simulink model "LQR"  (R2024a)
settings: Solver=ode4  StartTime=0.0  StopTime=simtime  FixedStep=0.1  RelTol=1e-3
values from neighbouring files (symbols this model uses):
  C = [1 0 0 0 0 0 -1 0 0 0 0 0 ... (45 elements, 5x9)]    [C.mat]
undefined symbols (not defined in the file or in its folder): Ki, Kp, syys
settings Model: Creator=soeta  LastModifiedBy=soeta
settings DataIOCC: ReturnWorkspaceOutputs=off

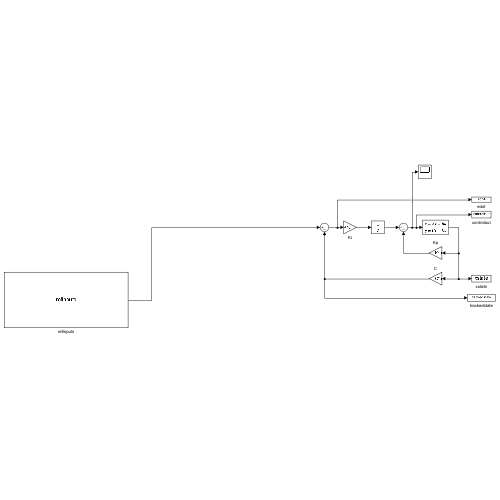
[thumbnail: Simulink's stored preview of the top-level diagram]
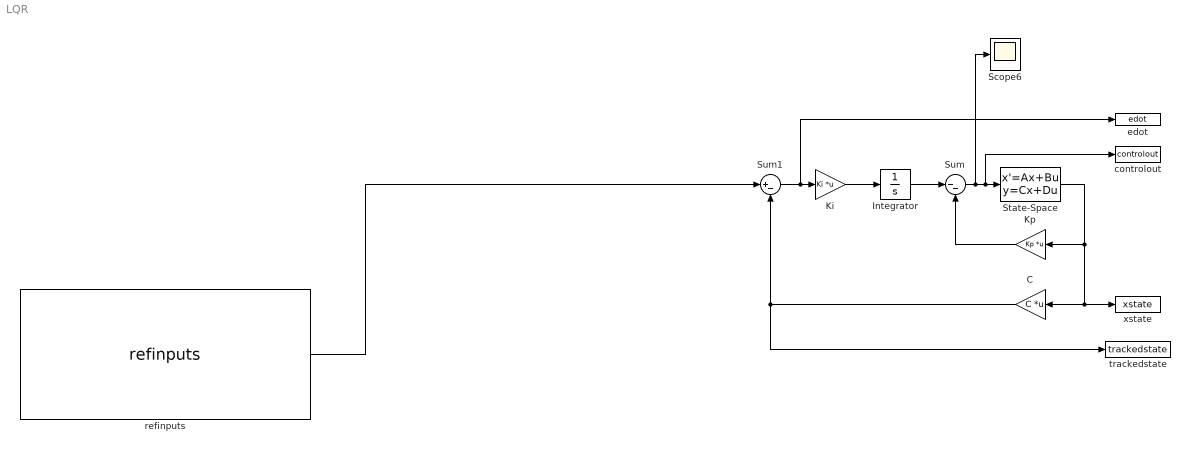
== system LQR ==
  C : Gain  Gain=C  Multiplication=Matrix(K*u)
  Integrator : Integrator
  Ki : Gain  Gain=Ki  Multiplication=Matrix(K*u)
  Kp : Gain  Gain=Kp  Multiplication=Matrix(K*u)
  Scope6 : Scope
  State-Space : StateSpace  A=syys.A  B=syys.B  C=syys.C  D=syys.D  InitialCondition=0
  Sum : Sum  Inputs=|--
  Sum1 : Sum  Inputs=|+-
  controlout : ToWorkspace  VariableName=controlout  SaveFormat=Timeseries  SampleTime=-1
  edot : ToWorkspace  VariableName=edot  SaveFormat=Timeseries  SampleTime=-1
  refinputs : FromWorkspace  VariableName=refinputs
  trackedstate : ToWorkspace  VariableName=trackedstate  SaveFormat=Timeseries  SampleTime=-1
  xstate : ToWorkspace  VariableName=xstate  SaveFormat=Timeseries  SampleTime=-1
  wires:
  Integrator/1 -> Sum/1
  State-Space/1 -> xstate/1, C/1, Kp/1
  Ki/1 -> Integrator/1
  C/1 -> trackedstate/1, Sum1/2
  refinputs/1 -> Sum1/1
  Kp/1 -> Sum/2
  Sum1/1 -> edot/1, Ki/1
  Sum/1 -> Scope6/1, controlout/1, State-Space/1
